simulink library "pwrsysVSrc"  (R2016a)
settings: Solver=VariableStepAuto  SolverMode=SingleTasking  StartTime=0.0  StopTime=10.0  RelTol=1e-3
undefined symbols (not defined in the file or in its folder): D1, Delta, DiscIntNeverNeededParam, ESS, fn, grid, Kp, PCC, Refmax, Refmin, sim, Tsm
undefined symbols (not defined in the file): exc, gov, Ts_c, turb, WT
libraries: powerlib x74, pwrsysBasic x1, sps_avr x1
settings Model: Creator=daniemot  LastModifiedBy=ericfa
settings DebuggingCC: SFUnexpectedBacktrackingDiag=error  SFNoUnconditionalDefaultTransitionDiag=error
settings GRTTargetCC: TargetLangStandard=C99 (ISO)  GeneratePreprocessorConditionals=Use local settings
settings ConfigComp: CovMetricSettings=dwe  CovHtmlReporting=off  CovSaveCumulativeToWorkspaceVar=off  CovSaveSingleToWorkspaceVar=off  CovExternalEMLEnable=on

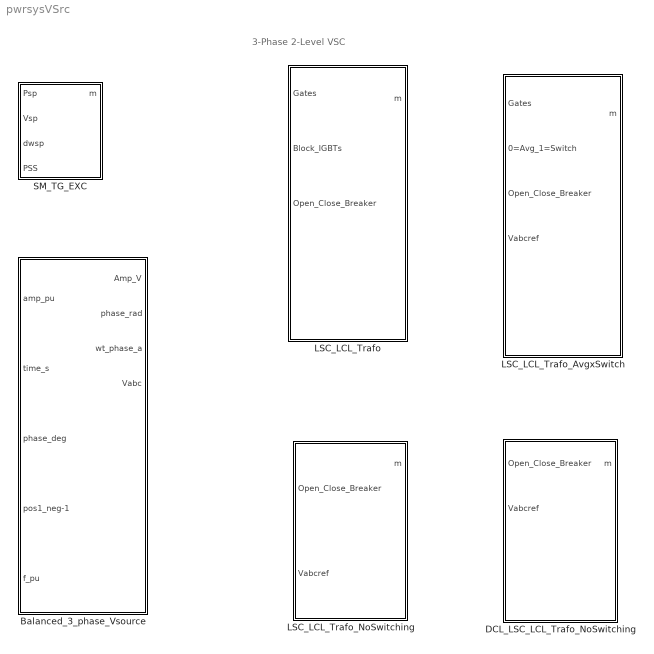
== system pwrsysVSrc ==
  note: 3-Phase 2-Level VSC
  Balanced_3_phase_Vsource : Subsystem  mask(Three-phase ideal voltage source){BaseAmp=1, fn=50}
      mask prompts: BaseAmp "Base phase-to-neutral amplitude [V]"; fn "Base frequency [Hz]"
      mask help:
      | Three-phase balanced ideal voltage source with neutral point not connected.
      | The voltage source can be connected in series with others.
      |
      | va [V] = amp_pu*BaseAmp*sin(2*pi*f_pu*fn*time + phase_deg*pi/180)
      | vb [V] = amp_pu*BaseAmp*sin(2*pi*f_pu*fn*time + phase_deg*pi/180 + Ph_b_sign*2*pi/3)
      | vc [V] = amp_pu*BaseAmp*sin(2*pi*f_pu*fn*time + phase_deg*pi/180 + Ph_c_sign*2*pi/3)
      |
      | If Pos1_Neg-1 = 1
      | 	Ph_b_sign = -1
      | 	Ph_c_sign = +1
      |
      | If Pos1_Neg-1 = -1
      | 	Ph_b_sign = +1
      | 	Ph_c_sign = -1
  DCL_LSC_LCL_Trafo_NoSwitching : Subsystem  mask(DCL + LSC + LCL + Trafo){Sn=WT.Sb, fn=fn, Uhv_ab=WT.ColSys.Ub, Uab=WT.LSC.Ub, lf2=WT.LSC.lf2, rf2=WT.LSC.rf2, Lf1=WT.LSC.Lf1, Rf1=WT.LSC.Rf1, Cf=WT.LSC.Cf, Rc=WT.LSC.Rc, Cdc=WT.LSC.Cf, Udc0=WT.LSC.Cf, Tsm=Tsm, Tstart=WT.LSC.Rc}
      mask prompts: Sn "Rated apparent power [VA]"; fn "Rated frequency [Hz]"; Uhv_ab "Trafo HV rated line voltage [V]"; Uab "Trafo LV rated line voltage [V]"; lf2 "Trafo short-circuit inductance, lf2 [pu]"; rf2 "Trafo short-circuit resistance, rf2 [pu]"; Lf1 "Inverter side inductande, Lf1 [H]"; Rf1 "Inverter side parasitic resistance, Rf1 [Ohm]"; Cf "Shunt branch capacitance, Cf [F]"; Rc "Shunt branch damping resistance, Rc [Ohm]"; Cdc "DC-link shunt capacitance, Cdc [F]"; Udc0 "DC-link initial voltage [V]"; Tsm "Measurement sampling time [s]"; Tstart "Start time [s]"
      mask help:
      | DC Link + Line-side converter + LCL filter + Transformer
      |
      | DCL: current sources
      | 	Cdc: shunt capacitor of DC-link
      |
      | LSC: voltage source
      | 	fpwm: PWM frequency
      | LCL:
      | 	Lf1 + Rf1: inverter side reactor
      | 	Cf + Rc: shunt capacitor and damping resistor
      | 	Lf2 + Rf2: transformer short circuit inductance and resistance
      |
      | Transformer:	Y d1
      | 	HV: Y ungrounded
      | 	LV: delta
      |
      | High resistive grounding on LV side of tranformer (0.001W)
  LSC_LCL_Trafo : Subsystem  mask(LSC + LCL + Trafo){Sn=WT.Sb, fn=fn, Uhv_ab=WT.ColSys.Ub, Uab=WT.LSC.Ub, lf2=WT.LSC.lf2, rf2=WT.LSC.rf2, Lf1=WT.LSC.Lf1, Rf1=WT.LSC.Rf1, Cf=WT.LSC.Cf, Rc=WT.LSC.Rc}
      mask prompts: Sn "Rated apparent power [VA]"; fn "Rated frequency [Hz]"; Uhv_ab "Trafo HV rated line voltage [V]"; Uab "Trafo LV rated line voltage [V]"; lf2 "Trafo short-circuit inductance, lf2 [pu]"; rf2 "Trafo short-circuit resistance, rf2 [pu]"; Lf1 "Inverter side inductande, Lf1 [H]"; Rf1 "Inverter side parasitic resistance, Rf1 [Ohm]"; Cf "Shunt branch capacitance, Cf [F]"; Rc "Shunt branch damping resistance, Rc [Ohm]"
      mask help:
      | Line side converter + LCL filter + Transformer
      |
      | LSC: switching devices
      | LCL:
      | 	Lf1 + Rf1: inverter side reactor
      | 	Cf + Rc: shunt capacitor and damping resistor
      | 	Lf2 + Rf2: transformer short circuit inductance and resistance
      |
      | Transformer:	Y d1
      | 	HV: Y ungrounded
      | 	LV: delta
      |
      | High resistive grounding on LV side of tranformer (0.001W)
  LSC_LCL_Trafo_AvgxSwitch : Subsystem  mask(LSC + LCL + Trafo){Sn=WT.Sb, fn=fn, Uhv_ab=WT.ColSys.Ub, Uab=WT.LSC.Ub, lf2=WT.LSC.lf2, rf2=WT.LSC.rf2, Lf1=WT.LSC.Lf1, Rf1=WT.LSC.Rf1, Cf=WT.LSC.Cf, Rc=WT.LSC.Rc}
      mask prompts: Sn "Rated apparent power [VA]"; fn "Rated frequency [Hz]"; Uhv_ab "Trafo HV rated line voltage [V]"; Uab "Trafo LV rated line voltage [V]"; lf2 "Trafo short-circuit inductance, lf2 [pu]"; rf2 "Trafo short-circuit resistance, rf2 [pu]"; Lf1 "Inverter side inductande, Lf1 [H]"; Rf1 "Inverter side parasitic resistance, Rf1 [Ohm]"; Cf "Shunt branch capacitance, Cf [F]"; Rc "Shunt branch damping resistance, Rc [Ohm]"
      mask help:
      | Line side converter + LCL filter + Transformer
      |
      | LSC: switching devices
      | LCL:
      | 	Lf1 + Rf1: inverter side reactor
      | 	Cf + Rc: shunt capacitor and damping resistor
      | 	Lf2 + Rf2: transformer short circuit inductance and resistance
      |
      | Transformer:	Y d1
      | 	HV: Y ungrounded
      | 	LV: delta
      |
      | High resistive grounding on LV side of tranformer (0.001W)
  LSC_LCL_Trafo_NoSwitching : Subsystem  mask(LSC + LCL + Trafo){Sn=WT.Sb, fn=fn, Uhv_ab=WT.ColSys.Ub, Uab=WT.LSC.Ub, lf2=WT.LSC.lf2, rf2=WT.LSC.rf2, Lf1=WT.LSC.Lf1, Rf1=WT.LSC.Rf1, Cf=WT.LSC.Cf, Rc=WT.LSC.Rc}
      mask prompts: Sn "Rated apparent power [VA]"; fn "Rated frequency [Hz]"; Uhv_ab "Trafo HV rated line voltage [V]"; Uab "Trafo LV rated line voltage [V]"; lf2 "Trafo short-circuit inductance, lf2 [pu]"; rf2 "Trafo short-circuit resistance, rf2 [pu]"; Lf1 "Inverter side inductande, Lf1 [H]"; Rf1 "Inverter side parasitic resistance, Rf1 [Ohm]"; Cf "Shunt branch capacitance, Cf [F]"; Rc "Shunt branch damping resistance, Rc [Ohm]"
      mask help:
      | Line side converter + LCL filter + Transformer
      |
      | LSC: switching devices
      | LCL:
      | 	Lf1 + Rf1: inverter side reactor
      | 	Cf + Rc: shunt capacitor and damping resistor
      | 	Lf2 + Rf2: transformer short circuit inductance and resistance
      |
      | Transformer:	Y d1
      | 	HV: Y ungrounded
      | 	LV: delta
      |
      | High resistive grounding on LV side of tranformer (0.001W)
  SM_TG_EXC : Subsystem  SystemSampleTime=10*sim.tStep  mask(Synchronous machine with governor and exciter){SMVn=sm.Vn, SMPn=sm.Sn, SMcosphi=sm.cosphi, SMfn=sm.fn, SMp=sm.p, SMM=sm.M, SMsat=sm.sat, SMXd=sm.Xd, SMXdp=sm.Xdp, SMXdpp=sm.Xdpp, SMXq=sm.Xq, SMXqpp=sm.Xqpp, SMXl=sm.Xl, SMRs=sm.Rs, SMTdpSC=sm.TdpSC, SMTdppSC=sm.TdppSC, SMTqppSC=sm.TqppSC, TurbT=turb.T, Ts=Ts_c, GovKp=gov.Kp, GovKd=gov.Kd, GovTr=gov.Tr, GovFlp=gov.flp, GovDB=gov.DB, ExcTr=exc.Tr, ExcKa=exc.Ka, ExcVRMax=exc.VRmax, ExcVRMin=exc.VRmin, ExcKf=exc.Kf, ExcTf=exc.Tf, ExcTb=exc.Tb, ExcTc=exc.Tc, ExcTb1=exc.Tb1, ExcTc1=exc.Tc1, TurbP0=turb.P0, SMVt0=sm.Vt0, SMEfd0=sm.Efd0, SMdw0=sm.dw0, SMth0=sm.th0, SMphi0=sm.phi0}
      mask prompts: SMVn "Voltage [V]"; SMPn "Apparent power [VA]"; SMcosphi "Power factor"; SMfn "Frequency [Hz]"; SMp "Pairs of poles"; SMM "Inertia constant [s]"; SMsat "Saturation curve in pu - [ifd; vt]"; SMXd "d-axis steady-state"; SMXdp "d-axis transient"; SMXdpp "d-axis subtransient"; SMXq "q-axis steady-state"; SMXqpp "q-axis subtransient"; SMXl "Leakage"; SMRs "Stator (armature) resistance"; SMTdpSC "d-axis transient time"; SMTdppSC "d-axis subtransient time"; SMTqppSC "q-axis subtransient time"; TurbT "Equivalent first-order delay [s]"; Ts "Sample time [s]"; GovKp "Permanent droop (primary control)"; GovKd "Transient droop (primary control)"; GovTr "Reset time transient droop (primary control)"; GovFlp "Low-pass frequency [Hz]"; GovDB "Deadband [pu]"; ExcTr "Input filter time constant [s]"; ExcKa "Proportional gain"; ExcVRMax "Maximum output [pu]"; ExcVRMin "Minimum output [pu]"; ExcKf "Rate feedback (derivative) gain"; ExcTf "Rate feedback (reset) time [s]"; ExcTb "1st lag time constant [s]"; ExcTc "1st lead time constant [s]"; ExcTb1 "2nd lag time constant [s]"; ExcTc1 "2nd lead time constant [s]"; TurbP0 "Turbine output [pu]"; SMVt0 "Stator voltage [pu]"; SMEfd0 "Field voltage [pu]"; SMdw0 "dw [%]"; SMth0 "theta [deg]"; SMphi0 "phi [deg]"
      mask help:
      | Synchronous machine + Generic Turbine Governor + IEEE ST1A Exciter
      |
      | This block is built using elements of the Simscape Specialized Power Systems library.
      |
      | Inputs:
      | Psp - Active power (P) setpoint in pu.
      |     Feed-forwarded to the turbine governor's Pxf droop controller. For precise P control, implement an external P controller.
      |
      | Vsp - RMS average voltage in pu.
      |     Connected to the Vref input of the IEEE ST1A Exciter.
      |
      | PSS - PSS contribution in pu.
      |     Connected to the Vstab input of the IEEE ST1A Exciter. Implement the PSS control loop externally.

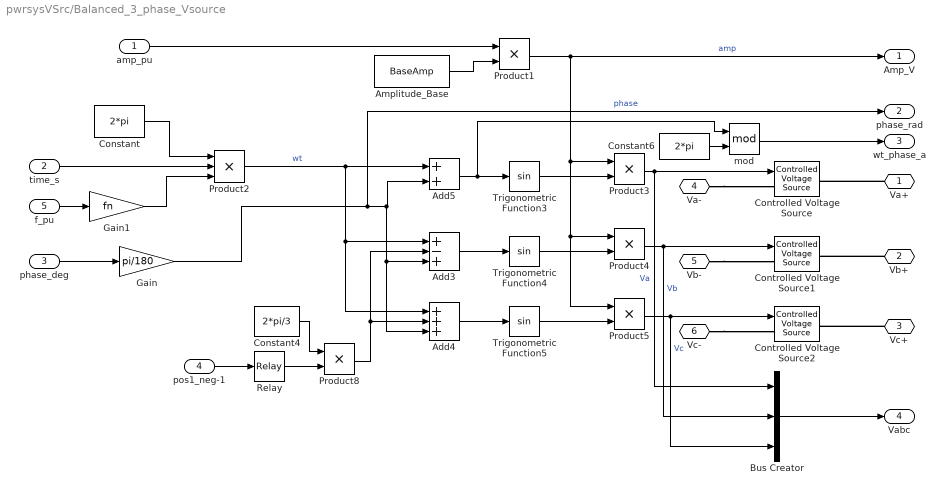
== system pwrsysVSrc/Balanced_3_phase_Vsource ==
  amp_pu : Inport
  time_s : Inport  Port=2
  phase_deg : Inport  Port=3
  pos1_neg-1 : Inport  Port=4
  f_pu : Inport  Port=5
  Add3 : Sum  Inputs=+-+
  Add4 : Sum  Inputs=+++
  Add5 : Sum
  Amplitude_Base : Constant  Value=BaseAmp
  Bus Creator : BusCreator  Inputs=3
  Constant : Constant  Value=2*pi
  Constant4 : Constant  Value=2*pi/3
  Constant6 : Constant  Value=2*pi
  Controlled Voltage Source : powerlib/Electrical Sources/Controlled Voltage Source  Initialize=off  Source_Type=AC  Amplitude=ESS.LSC.Ub*(2/3)^0.5  Phase=0  Frequency=PCC.fn  Measurements=None
  Controlled Voltage Source1 : powerlib/Electrical Sources/Controlled Voltage Source  Initialize=off  Source_Type=AC  Amplitude=ESS.LSC.Ub*(2/3)^0.5  Phase=-120  Frequency=PCC.fn  Measurements=None
  Controlled Voltage Source2 : powerlib/Electrical Sources/Controlled Voltage Source  Initialize=off  Source_Type=AC  Amplitude=ESS.LSC.Ub*(2/3)^0.5  Phase=120  Frequency=PCC.fn  Measurements=None
  Gain : Gain  Gain=pi/180
  Gain1 : Gain  Gain=fn
  Product{1,3..5,8} (5 alike) : Product
  Product2 : Product  Inputs=3
  Relay : Relay  OnSwitchValue=0  OffSwitchValue=-0.1  OffOutputValue=-1
  Trigonometric Function3 : Trigonometry
  Trigonometric Function4 : Trigonometry
  Trigonometric Function5 : Trigonometry
  mod : Math  Operator=mod  SaturateOnIntegerOverflow=on
  Va+ : PMIOPort  Port=1  Side=Right
  Vb+ : PMIOPort  Port=2  Side=Right
  Vc+ : PMIOPort  Port=3  Side=Right
  Va- : PMIOPort  Port=4  Side=Right
  Vb- : PMIOPort  Port=5  Side=Right
  Vc- : PMIOPort  Port=6  Side=Right
  Amp_V : Outport
  phase_rad : Outport  Port=2
  wt_phase_a : Outport  Port=3
  Vabc : Outport  Port=4
  wires:
  Add4/1 -> Trigonometric Function5/1
  Gain/1 -> phase_rad/1, Add4/3, Add3/3, Add5/2  "phase"
  Add3/1 -> Trigonometric Function4/1
  pos1_neg-1/1 -> Relay/1
  Product3/1 -> Bus Creator/1, Controlled Voltage Source/1  "Va"
  amp_pu/1 -> Product1/1
  Product8/1 -> Add3/2, Add4/2
  Product5/1 -> Bus Creator/3, Controlled Voltage Source2/1  "Vc"
  Product4/1 -> Bus Creator/2, Controlled Voltage Source1/1  "Vb"
  Amplitude_Base/1 -> Product1/2
  Constant4/1 -> Product8/1
  Product1/1 -> Product5/1, Product4/1, Product3/1, Amp_V/1  "amp"
  Relay/1 -> Product8/2
  Trigonometric Function3/1 -> Product3/2
  Product2/1 -> Add5/1, Add4/1, Add3/1  "wt"
  Trigonometric Function5/1 -> Product5/2
  Add5/1 -> mod/1, Trigonometric Function3/1
  Trigonometric Function4/1 -> Product4/2
  phase_deg/1 -> Gain/1
  time_s/1 -> Product2/2
  Constant/1 -> Product2/1
  f_pu/1 -> Gain1/1
  Gain1/1 -> Product2/3
  Bus Creator/1 -> Vabc/1
  Constant6/1 -> mod/2
  mod/1 -> wt_phase_a/1
  connections:
  Vb+/RConn1 -- Controlled Voltage Source1/RConn1
  Vc+/RConn1 -- Controlled Voltage Source2/RConn1
  Va+/RConn1 -- Controlled Voltage Source/RConn1
  Va-/RConn1 -- Controlled Voltage Source/LConn1
  Vb-/RConn1 -- Controlled Voltage Source1/LConn1
  Vc-/RConn1 -- Controlled Voltage Source2/LConn1

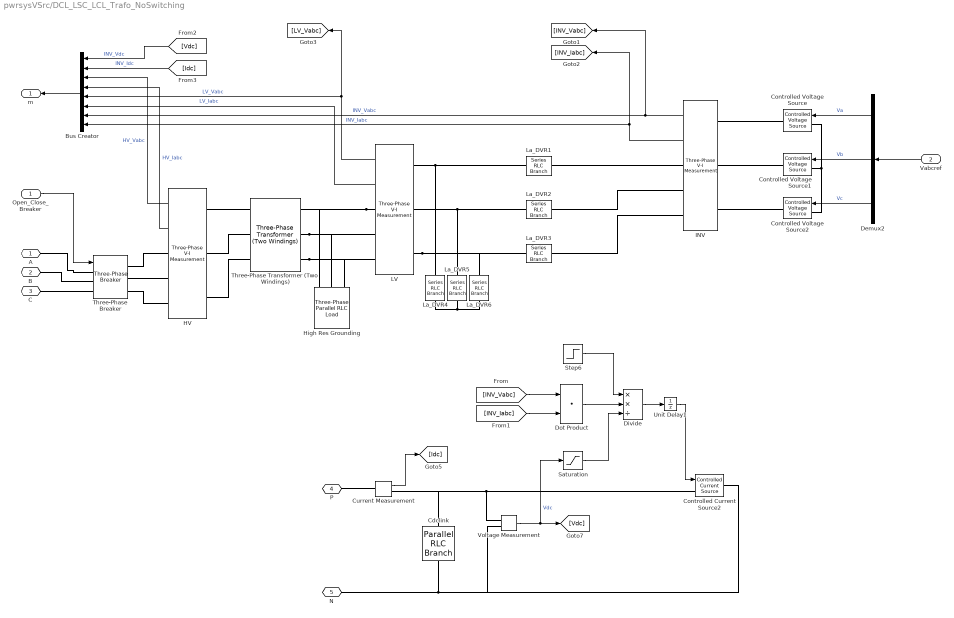
== system pwrsysVSrc/DCL_LSC_LCL_Trafo_NoSwitching ==
  Open_Close_Breaker : Inport
  Vabcref : Inport  Port=2
  Bus Creator : BusCreator  Inputs=8
  Cdclink : powerlib/Elements/Parallel RLC Branch  LConnTagsString=a  RConnTagsString=__new0  BranchType=RC  Resistance=1e6  Inductance=0  SetiL0=off  InitialCurrent=0  Capacitance=Cdc  Setx0=on  InitialVoltage=Udc0  Measurements=None
  Controlled Current Source2 : powerlib/Electrical Sources/Controlled Current Source  Initialize=on  Source_Type=DC  Amplitude=0  Phase=0  Frequency=50  Measurements=None
  Controlled Voltage Source : powerlib/Electrical Sources/Controlled Voltage Source  Initialize=on  Source_Type=AC  Amplitude=Uab*(2/3)^0.5  Phase=30  Frequency=fn  Measurements=None
  Controlled Voltage Source1 : powerlib/Electrical Sources/Controlled Voltage Source  Initialize=on  Source_Type=AC  Amplitude=Uab*(2/3)^0.5  Phase=30-120  Frequency=fn  Measurements=None
  Controlled Voltage Source2 : powerlib/Electrical Sources/Controlled Voltage Source  Initialize=on  Source_Type=AC  Amplitude=Uab*(2/3)^0.5  Phase=30+120  Frequency=fn  Measurements=None
  Current Measurement : powerlib/Measurements/Current Measurement  PhasorSimulation=off  OutputType=Complex  PSBequivalent=0
  Demux2 : Demux  Outputs=3
  Divide : Product  Inputs=**/
  Dot Product : DotProduct  InputSameDT=on  OutDataTypeStr=Inherit: Inherit via internal rule
  HV : powerlib/Measurements/Three-Phase V-I Measurement  VoltageMeasurement=phase-to-ground  SetLabelV=off  LabelV=vgrid  Vpu=off  VpuLL=off  CurrentMeasurement=yes  SetLabelI=off  LabelI=igrid  Ipu=off  Pbase=sn  Vbase=uab  OutputType=Complex  PhasorSimulation=off  PSBequivalent=0
  High Res Grounding : powerlib/Elements/Three-Phase Parallel RLC Load  LConnTagsString=A|B|C  Configuration=Y (grounded)  NominalVoltage=Uab  Vabc=[1e3 1e3 1e3]  Vabcp=[1e3 1e3 1e3]  NominalFrequency=fn  UnbalancedPower=off  ActivePower=0.001  InductivePower=0  CapacitivePower=0  Pabc=[10e3 9e3 11e3]  QLabc=[100 90 110]  QCabc=[100 90 110]  Pabcp=[10e3 9e3 11e3]  QLabcp=[100 90 110]  QCabcp=[100 90 110]  Measurements=None  LoadType=constant Z
  INV : powerlib/Measurements/Three-Phase V-I Measurement  VoltageMeasurement=phase-to-ground  SetLabelV=off  LabelV=vconv  Vpu=off  VpuLL=off  CurrentMeasurement=yes  SetLabelI=off  LabelI=iconv  Ipu=off  Pbase=sn  Vbase=uab  OutputType=Complex  PhasorSimulation=off  PSBequivalent=0
  LV : powerlib/Measurements/Three-Phase V-I Measurement  VoltageMeasurement=phase-to-ground  SetLabelV=off  LabelV=vgrid  Vpu=off  VpuLL=off  CurrentMeasurement=yes  SetLabelI=off  LabelI=igrid  Ipu=off  Pbase=sn  Vbase=uab  OutputType=Complex  PhasorSimulation=off  PSBequivalent=0
  La_DVR1 : powerlib/Elements/Series RLC Branch  LConnTagsString=__new0  RConnTagsString=__new0  BranchType=RL  Resistance=Rf1  Inductance=Lf1  SetiL0=off  InitialCurrent=0  Capacitance=1.0  Setx0=off  InitialVoltage=0  Measurements=None
  La_DVR2 : powerlib/Elements/Series RLC Branch  LConnTagsString=__new0  RConnTagsString=__new0  BranchType=RL  Resistance=Rf1  Inductance=Lf1  SetiL0=off  InitialCurrent=0  Capacitance=1.0  Setx0=off  InitialVoltage=0  Measurements=None
  La_DVR3 : powerlib/Elements/Series RLC Branch  LConnTagsString=__new0  RConnTagsString=__new0  BranchType=RL  Resistance=Rf1  Inductance=Lf1  SetiL0=off  InitialCurrent=0  Capacitance=1.0  Setx0=off  InitialVoltage=0  Measurements=None
  La_DVR4 : powerlib/Elements/Series RLC Branch  LConnTagsString=__new0  RConnTagsString=__new0  BranchType=RC  Resistance=Rc  Inductance=Lf1  SetiL0=off  InitialCurrent=0  Capacitance=Cf  Setx0=off  InitialVoltage=0  Measurements=None
  La_DVR5 : powerlib/Elements/Series RLC Branch  LConnTagsString=__new0  RConnTagsString=__new0  BranchType=RC  Resistance=Rc  Inductance=Lf1  SetiL0=off  InitialCurrent=0  Capacitance=Cf  Setx0=off  InitialVoltage=0  Measurements=None
  La_DVR6 : powerlib/Elements/Series RLC Branch  LConnTagsString=__new0  RConnTagsString=__new0  BranchType=RC  Resistance=Rc  Inductance=Lf1  SetiL0=off  InitialCurrent=0  Capacitance=Cf  Setx0=off  InitialVoltage=0  Measurements=None
  Saturation : Saturate  UpperLimit=10*Uab*sqrt(2/3)  LowerLimit=0.01*Uab*sqrt(2/3)
  Step6 : Step  Time=Tstart  SampleTime=Tsm
  Three-Phase Transformer (Two Windings) : powerlib/Elements/Three-Phase Transformer (Two Windings)  Winding1Connection=Y  Winding2Connection=Delta (D1)  CoreType=Three-limb core (core-type)  SetSaturation=off  Hysteresis=off  DataFile='hysteresis'  SetInitialFlux=off  Measurements=None  UNITS=pu  NominalPower=[ Sn , fn ]  Winding1=[ Uhv_ab , rf2/2 , lf2/2 ]  Winding2=[ Uab , rf2/2 , lf2/2 ]  Rm=500  Lm=500  L0=0.5  Saturation=[ 0,0 ; 0.0024,1.2 ; 1.0,1.52 ]  InitialFluxes=[0 0 0]  MoreParameters=off  BreakLoop=off  DataType=off  TransfoNumber=1
  Three-Phase Breaker : powerlib/Elements/Three-Phase Breaker  InitialState=open  SwitchA=on  SwitchB=on  SwitchC=on  SwitchTimes="[1/60  5/60]"  External=on  BreakerResistance=0.01  SnubberResistance=1e6  SnubberCapacitance=1e9  Measurements=None
  Unit Delay1 : UnitDelay  SampleTime=Tsm
  Voltage Measurement : powerlib/Measurements/Voltage Measurement  PhasorSimulation=off  OutputType=Magnitude  PSBequivalent=0
  A : PMIOPort  Port=1  Side=Right
  B : PMIOPort  Port=2  Side=Right
  C : PMIOPort  Port=3  Side=Right
  P : PMIOPort  Port=4  Side=Left
  N : PMIOPort  Port=5  Side=Left
  m : Outport
  wires:
  HV/2 -> Bus Creator/4  "HV_Iabc"
  LV/1 -> [LV_Vabc], Bus Creator/5  "LV_Vabc"
  INV/1 -> [INV_Vabc], Bus Creator/7  "INV_Vabc"
  INV/2 -> [INV_Iabc], Bus Creator/8  "INV_Iabc"
  HV/1 -> Bus Creator/3  "HV_Vabc"
  LV/2 -> Bus Creator/6  "LV_Iabc"
  Bus Creator/1 -> m/1
  Open_Close_Breaker/1 -> Three-Phase Breaker/1
  Vabcref/1 -> Demux2/1
  Demux2/1 -> Controlled Voltage Source/1  "Va"
  Demux2/2 -> Controlled Voltage Source1/1  "Vb"
  Demux2/3 -> Controlled Voltage Source2/1  "Vc"
  Voltage Measurement/1 -> [Vdc], Saturation/1  "Vdc"
  Saturation/1 -> Divide/3
  Dot Product/1 -> Divide/2
  Divide/1 -> Unit Delay1/1
  [INV_Vabc] -> Dot Product/1
  [INV_Iabc] -> Dot Product/2
  [Vdc] -> Bus Creator/1  "INV_Vdc"
  [Idc] -> Bus Creator/2  "INV_Idc"
  Unit Delay1/1 -> Controlled Current Source2/1
  Step6/1 -> Divide/1
  Current Measurement/1 -> [Idc]
  connections:
  La_DVR1/LConn1 -- INV/RConn1
  LV/RConn1 -- Three-Phase Transformer (Two Windings)/RConn1 -- High Res Grounding/LConn1
  La_DVR1/RConn1 -- La_DVR4/RConn1 -- LV/LConn1
  Three-Phase Transformer (Two Windings)/LConn3 -- HV/LConn3
  Three-Phase Transformer (Two Windings)/RConn3 -- LV/RConn3 -- High Res Grounding/LConn3
  La_DVR2/RConn1 -- La_DVR5/RConn1 -- LV/LConn2
  Three-Phase Transformer (Two Windings)/LConn2 -- HV/LConn2
  Three-Phase Transformer (Two Windings)/RConn2 -- LV/RConn2 -- High Res Grounding/LConn2
  Three-Phase Transformer (Two Windings)/LConn1 -- HV/LConn1
  LV/LConn3 -- La_DVR3/RConn1 -- La_DVR6/RConn1
  La_DVR3/LConn1 -- INV/RConn3
  La_DVR5/LConn1 -- La_DVR6/LConn1 -- La_DVR4/LConn1
  La_DVR2/LConn1 -- INV/RConn2
  Three-Phase Breaker/LConn2 -- B/RConn1
  Three-Phase Breaker/RConn2 -- HV/RConn2
  HV/RConn3 -- Three-Phase Breaker/RConn3
  Three-Phase Breaker/LConn3 -- C/RConn1
  HV/RConn1 -- Three-Phase Breaker/RConn1
  Three-Phase Breaker/LConn1 -- A/RConn1
  Controlled Voltage Source2/LConn1 -- Controlled Voltage Source/LConn1 -- Controlled Voltage Source1/LConn1
  INV/LConn1 -- Controlled Voltage Source/RConn1
  Controlled Voltage Source1/RConn1 -- INV/LConn2
  Controlled Voltage Source2/RConn1 -- INV/LConn3
  Voltage Measurement/LConn2 -- Controlled Current Source2/RConn1 -- Cdclink/RConn1 -- N/RConn1
  Controlled Current Source2/LConn1 -- Current Measurement/RConn1 -- Cdclink/LConn1 -- Voltage Measurement/LConn1
  P/RConn1 -- Current Measurement/LConn1

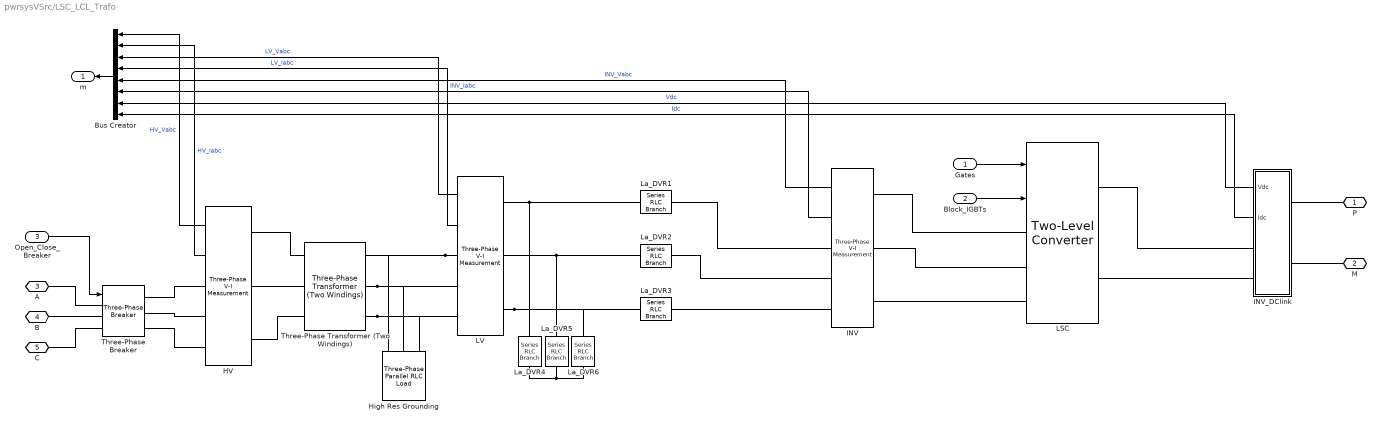
== system pwrsysVSrc/LSC_LCL_Trafo ==
  Gates : Inport
  Block_IGBTs : Inport  Port=2
  Open_Close_Breaker : Inport  Port=3
  Bus Creator : BusCreator  Inputs=8
  HV : powerlib/Measurements/Three-Phase V-I Measurement  VoltageMeasurement=phase-to-ground  SetLabelV=off  LabelV=vgrid  Vpu=off  VpuLL=off  CurrentMeasurement=yes  SetLabelI=off  LabelI=igrid  Ipu=off  Pbase=sn  Vbase=uab  OutputType=Complex  PhasorSimulation=off  PSBequivalent=0
  High Res Grounding : powerlib/Elements/Three-Phase Parallel RLC Load  LConnTagsString=A|B|C  Configuration=Y (grounded)  NominalVoltage=Uab  Vabc=[1e3 1e3 1e3]  Vabcp=[1e3 1e3 1e3]  NominalFrequency=fn  UnbalancedPower=off  ActivePower=0.001  InductivePower=0  CapacitivePower=0  Pabc=[10e3 9e3 11e3]  QLabc=[100 90 110]  QCabc=[100 90 110]  Pabcp=[10e3 9e3 11e3]  QLabcp=[100 90 110]  QCabcp=[100 90 110]  Measurements=None  LoadType=constant Z
  INV : powerlib/Measurements/Three-Phase V-I Measurement  VoltageMeasurement=phase-to-ground  SetLabelV=off  LabelV=vconv  Vpu=off  VpuLL=off  CurrentMeasurement=yes  SetLabelI=off  LabelI=iconv  Ipu=off  Pbase=sn  Vbase=uab  OutputType=Complex  PhasorSimulation=off  PSBequivalent=0
  INV_DClink : Subsystem
  LSC : powerlib/Power Electronics/Two-Level Converter  ModelType=Switching devices  Ron=1e-3  Rs=1e6  Cs=inf  Vforward=[ 0, 0 ]  Ron_Diode=1e-3  Rs_Diode=1e6  Cs_Diode=inf  Vf_Diode=1e-3  Rs_CurrentSource=inf
      settings: AttributesFormatString=%<ModelType>
  LV : powerlib/Measurements/Three-Phase V-I Measurement  VoltageMeasurement=phase-to-ground  SetLabelV=off  LabelV=vgrid  Vpu=off  VpuLL=off  CurrentMeasurement=yes  SetLabelI=off  LabelI=igrid  Ipu=off  Pbase=sn  Vbase=uab  OutputType=Complex  PhasorSimulation=off  PSBequivalent=0
  La_DVR1 : powerlib/Elements/Series RLC Branch  LConnTagsString=__new0  RConnTagsString=__new0  BranchType=RL  Resistance=Rf1  Inductance=Lf1  SetiL0=off  InitialCurrent=0  Capacitance=1.0  Setx0=off  InitialVoltage=0  Measurements=None
  La_DVR2 : powerlib/Elements/Series RLC Branch  LConnTagsString=__new0  RConnTagsString=__new0  BranchType=RL  Resistance=Rf1  Inductance=Lf1  SetiL0=off  InitialCurrent=0  Capacitance=1.0  Setx0=off  InitialVoltage=0  Measurements=None
  La_DVR3 : powerlib/Elements/Series RLC Branch  LConnTagsString=__new0  RConnTagsString=__new0  BranchType=RL  Resistance=Rf1  Inductance=Lf1  SetiL0=off  InitialCurrent=0  Capacitance=1.0  Setx0=off  InitialVoltage=0  Measurements=None
  La_DVR4 : powerlib/Elements/Series RLC Branch  LConnTagsString=__new0  RConnTagsString=__new0  BranchType=RC  Resistance=Rc  Inductance=Lf1  SetiL0=off  InitialCurrent=0  Capacitance=Cf  Setx0=off  InitialVoltage=0  Measurements=None
  La_DVR5 : powerlib/Elements/Series RLC Branch  LConnTagsString=__new0  RConnTagsString=__new0  BranchType=RC  Resistance=Rc  Inductance=Lf1  SetiL0=off  InitialCurrent=0  Capacitance=Cf  Setx0=off  InitialVoltage=0  Measurements=None
  La_DVR6 : powerlib/Elements/Series RLC Branch  LConnTagsString=__new0  RConnTagsString=__new0  BranchType=RC  Resistance=Rc  Inductance=Lf1  SetiL0=off  InitialCurrent=0  Capacitance=Cf  Setx0=off  InitialVoltage=0  Measurements=None
  Three-Phase Transformer (Two Windings) : powerlib/Elements/Three-Phase Transformer (Two Windings)  Winding1Connection=Y  Winding2Connection=Delta (D1)  CoreType=Three-limb core (core-type)  SetSaturation=off  Hysteresis=off  DataFile='hysteresis'  SetInitialFlux=off  Measurements=None  UNITS=pu  NominalPower=[ Sn , fn ]  Winding1=[ Uhv_ab , rf2/2 , lf2/2 ]  Winding2=[ Uab , rf2/2 , lf2/2 ]  Rm=500  Lm=500  L0=0.5  Saturation=[ 0,0 ; 0.0024,1.2 ; 1.0,1.52 ]  InitialFluxes=[0 0 0]  MoreParameters=off  BreakLoop=off  DataType=off  TransfoNumber=1
  Three-Phase Breaker : powerlib/Elements/Three-Phase Breaker  InitialState=open  SwitchA=on  SwitchB=on  SwitchC=on  SwitchTimes="[1/60  5/60]"  External=on  BreakerResistance=0.01  SnubberResistance=1e6  SnubberCapacitance=1e9  Measurements=None
  "\tP" : PMIOPort  Port=1  Side=Left
  M : PMIOPort  Port=2  Side=Left
  A : PMIOPort  Port=3  Side=Right
  B : PMIOPort  Port=4  Side=Right
  C : PMIOPort  Port=5  Side=Right
  m : Outport
  wires:
  HV/2 -> Bus Creator/2  "HV_Iabc"
  LV/1 -> Bus Creator/3  "LV_Vabc"
  INV/1 -> Bus Creator/5  "INV_Vabc"
  INV_DClink/2(Idc) -> Bus Creator/8  "Idc"
  INV/2 -> Bus Creator/6  "INV_Iabc"
  Block_IGBTs/1 -> LSC/2
  INV_DClink/1(Vdc) -> Bus Creator/7  "Vdc"
  HV/1 -> Bus Creator/1  "HV_Vabc"
  LV/2 -> Bus Creator/4  "LV_Iabc"
  Bus Creator/1 -> m/1
  Gates/1 -> LSC/1
  Open_Close_Breaker/1 -> Three-Phase Breaker/1
  connections:
  La_DVR1/LConn1 -- INV/RConn1
  LV/RConn1 -- Three-Phase Transformer (Two Windings)/RConn1 -- High Res Grounding/LConn1
  La_DVR1/RConn1 -- La_DVR4/RConn1 -- LV/LConn1
  LSC/LConn3 -- INV/LConn3
  Three-Phase Transformer (Two Windings)/LConn3 -- HV/LConn3
  LSC/LConn2 -- INV/LConn2
  Three-Phase Transformer (Two Windings)/RConn3 -- LV/RConn3 -- High Res Grounding/LConn3
  La_DVR2/RConn1 -- La_DVR5/RConn1 -- LV/LConn2
  Three-Phase Transformer (Two Windings)/LConn2 -- HV/LConn2
  LSC/RConn2 -- INV_DClink/RConn2
  LSC/LConn1 -- INV/LConn1
  LSC/RConn1 -- INV_DClink/RConn1
  Three-Phase Transformer (Two Windings)/RConn2 -- LV/RConn2 -- High Res Grounding/LConn2
  "\tP"/RConn1 -- INV_DClink/LConn1
  Three-Phase Transformer (Two Windings)/LConn1 -- HV/LConn1
  LV/LConn3 -- La_DVR3/RConn1 -- La_DVR6/RConn1
  La_DVR3/LConn1 -- INV/RConn3
  La_DVR5/LConn1 -- La_DVR6/LConn1 -- La_DVR4/LConn1
  La_DVR2/LConn1 -- INV/RConn2
  INV_DClink/LConn2 -- M/RConn1
  Three-Phase Breaker/LConn2 -- B/RConn1
  Three-Phase Breaker/RConn2 -- HV/RConn2
  HV/RConn3 -- Three-Phase Breaker/RConn3
  Three-Phase Breaker/LConn3 -- C/RConn1
  HV/RConn1 -- Three-Phase Breaker/RConn1
  Three-Phase Breaker/LConn1 -- A/RConn1

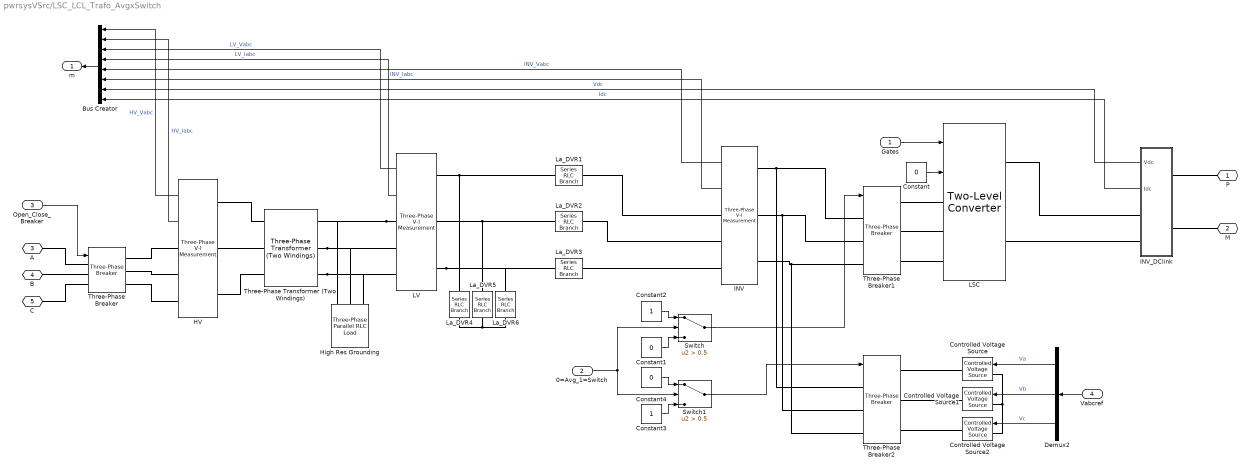
== system pwrsysVSrc/LSC_LCL_Trafo_AvgxSwitch ==
  Gates : Inport
  0=Avg_1=Switch : Inport  Port=2
  Open_Close_Breaker : Inport  Port=3
  Vabcref : Inport  Port=4
  Bus Creator : BusCreator  Inputs=8
  Constant : Constant  Value=0
  Constant1 : Constant  Value=0
  Constant2 : Constant
  Constant3 : Constant
  Constant4 : Constant  Value=0
  Controlled Voltage Source : powerlib/Electrical Sources/Controlled Voltage Source  Initialize=off  Source_Type=AC  Amplitude=ESS.LSC.Ub*(2/3)^0.5  Phase=0  Frequency=PCC.fn  Measurements=None
  Controlled Voltage Source1 : powerlib/Electrical Sources/Controlled Voltage Source  Initialize=off  Source_Type=AC  Amplitude=ESS.LSC.Ub*(2/3)^0.5  Phase=-120  Frequency=PCC.fn  Measurements=None
  Controlled Voltage Source2 : powerlib/Electrical Sources/Controlled Voltage Source  Initialize=off  Source_Type=AC  Amplitude=ESS.LSC.Ub*(2/3)^0.5  Phase=120  Frequency=PCC.fn  Measurements=None
  Demux2 : Demux  Outputs=3
  HV : powerlib/Measurements/Three-Phase V-I Measurement  VoltageMeasurement=phase-to-ground  SetLabelV=off  LabelV=vgrid  Vpu=off  VpuLL=off  CurrentMeasurement=yes  SetLabelI=off  LabelI=igrid  Ipu=off  Pbase=sn  Vbase=uab  OutputType=Complex  PhasorSimulation=off  PSBequivalent=0
  High Res Grounding : powerlib/Elements/Three-Phase Parallel RLC Load  LConnTagsString=A|B|C  Configuration=Y (grounded)  NominalVoltage=Uab  Vabc=[1e3 1e3 1e3]  Vabcp=[1e3 1e3 1e3]  NominalFrequency=fn  UnbalancedPower=off  ActivePower=0.001  InductivePower=0  CapacitivePower=0  Pabc=[10e3 9e3 11e3]  QLabc=[100 90 110]  QCabc=[100 90 110]  Pabcp=[10e3 9e3 11e3]  QLabcp=[100 90 110]  QCabcp=[100 90 110]  Measurements=None  LoadType=constant Z
  INV : powerlib/Measurements/Three-Phase V-I Measurement  VoltageMeasurement=phase-to-ground  SetLabelV=off  LabelV=vconv  Vpu=off  VpuLL=off  CurrentMeasurement=yes  SetLabelI=off  LabelI=iconv  Ipu=off  Pbase=sn  Vbase=uab  OutputType=Complex  PhasorSimulation=off  PSBequivalent=0
  INV_DClink : Subsystem
  LSC : powerlib/Power Electronics/Two-Level Converter  ModelType=Switching devices  Ron=1e-3  Rs=1e6  Cs=inf  Vforward=[ 0, 0 ]  Ron_Diode=1e-3  Rs_Diode=1e6  Cs_Diode=inf  Vf_Diode=1e-3  Rs_CurrentSource=inf
      settings: AttributesFormatString=%<ModelType>
  LV : powerlib/Measurements/Three-Phase V-I Measurement  VoltageMeasurement=phase-to-ground  SetLabelV=off  LabelV=vgrid  Vpu=off  VpuLL=off  CurrentMeasurement=yes  SetLabelI=off  LabelI=igrid  Ipu=off  Pbase=sn  Vbase=uab  OutputType=Complex  PhasorSimulation=off  PSBequivalent=0
  La_DVR1 : powerlib/Elements/Series RLC Branch  LConnTagsString=__new0  RConnTagsString=__new0  BranchType=RL  Resistance=Rf1  Inductance=Lf1  SetiL0=off  InitialCurrent=0  Capacitance=1.0  Setx0=off  InitialVoltage=0  Measurements=None
  La_DVR2 : powerlib/Elements/Series RLC Branch  LConnTagsString=__new0  RConnTagsString=__new0  BranchType=RL  Resistance=Rf1  Inductance=Lf1  SetiL0=off  InitialCurrent=0  Capacitance=1.0  Setx0=off  InitialVoltage=0  Measurements=None
  La_DVR3 : powerlib/Elements/Series RLC Branch  LConnTagsString=__new0  RConnTagsString=__new0  BranchType=RL  Resistance=Rf1  Inductance=Lf1  SetiL0=off  InitialCurrent=0  Capacitance=1.0  Setx0=off  InitialVoltage=0  Measurements=None
  La_DVR4 : powerlib/Elements/Series RLC Branch  LConnTagsString=__new0  RConnTagsString=__new0  BranchType=RC  Resistance=Rc  Inductance=Lf1  SetiL0=off  InitialCurrent=0  Capacitance=Cf  Setx0=off  InitialVoltage=0  Measurements=None
  La_DVR5 : powerlib/Elements/Series RLC Branch  LConnTagsString=__new0  RConnTagsString=__new0  BranchType=RC  Resistance=Rc  Inductance=Lf1  SetiL0=off  InitialCurrent=0  Capacitance=Cf  Setx0=off  InitialVoltage=0  Measurements=None
  La_DVR6 : powerlib/Elements/Series RLC Branch  LConnTagsString=__new0  RConnTagsString=__new0  BranchType=RC  Resistance=Rc  Inductance=Lf1  SetiL0=off  InitialCurrent=0  Capacitance=Cf  Setx0=off  InitialVoltage=0  Measurements=None
  Switch : Switch  Criteria=u2 > Threshold  Threshold=0.5
  Switch1 : Switch  Criteria=u2 > Threshold  Threshold=0.5
  Three-Phase Transformer (Two Windings) : powerlib/Elements/Three-Phase Transformer (Two Windings)  Winding1Connection=Y  Winding2Connection=Delta (D1)  CoreType=Three-limb core (core-type)  SetSaturation=off  Hysteresis=off  DataFile='hysteresis'  SetInitialFlux=off  Measurements=None  UNITS=pu  NominalPower=[ Sn , fn ]  Winding1=[ Uhv_ab , rf2/2 , lf2/2 ]  Winding2=[ Uab , rf2/2 , lf2/2 ]  Rm=500  Lm=500  L0=0.5  Saturation=[ 0,0 ; 0.0024,1.2 ; 1.0,1.52 ]  InitialFluxes=[0 0 0]  MoreParameters=off  BreakLoop=off  DataType=off  TransfoNumber=1
  Three-Phase Breaker : powerlib/Elements/Three-Phase Breaker  InitialState=open  SwitchA=on  SwitchB=on  SwitchC=on  SwitchTimes="[1/60  5/60]"  External=on  BreakerResistance=0.01  SnubberResistance=1e6  SnubberCapacitance=1e9  Measurements=None
  Three-Phase Breaker1 : powerlib/Elements/Three-Phase Breaker  InitialState=open  SwitchA=on  SwitchB=on  SwitchC=on  SwitchTimes="[1/60  5/60]"  External=on  BreakerResistance=0.000000000001  SnubberResistance=1e10  SnubberCapacitance=inf  Measurements=None
  Three-Phase Breaker2 : powerlib/Elements/Three-Phase Breaker  InitialState=open  SwitchA=on  SwitchB=on  SwitchC=on  SwitchTimes="[1/60  5/60]"  External=on  BreakerResistance=0.000000000001  SnubberResistance=1e10  SnubberCapacitance=inf  Measurements=None
  "\tP" : PMIOPort  Port=1  Side=Left
  M : PMIOPort  Port=2  Side=Left
  A : PMIOPort  Port=3  Side=Right
  B : PMIOPort  Port=4  Side=Right
  C : PMIOPort  Port=5  Side=Right
  m : Outport
  wires:
  HV/2 -> Bus Creator/2  "HV_Iabc"
  LV/1 -> Bus Creator/3  "LV_Vabc"
  INV/1 -> Bus Creator/5  "INV_Vabc"
  INV_DClink/2(Idc) -> Bus Creator/8  "Idc"
  INV/2 -> Bus Creator/6  "INV_Iabc"
  INV_DClink/1(Vdc) -> Bus Creator/7  "Vdc"
  HV/1 -> Bus Creator/1  "HV_Vabc"
  LV/2 -> Bus Creator/4  "LV_Iabc"
  Bus Creator/1 -> m/1
  Gates/1 -> LSC/1
  Open_Close_Breaker/1 -> Three-Phase Breaker/1
  Vabcref/1 -> Demux2/1
  Demux2/1 -> Controlled Voltage Source/1  "Va"
  Demux2/2 -> Controlled Voltage Source1/1  "Vb"
  Demux2/3 -> Controlled Voltage Source2/1  "Vc"
  Constant/1 -> LSC/2
  Constant1/1 -> Switch/3
  Constant2/1 -> Switch/1
  Switch/1 -> Three-Phase Breaker1/1
  Constant4/1 -> Switch1/1
  Constant3/1 -> Switch1/3
  Switch1/1 -> Three-Phase Breaker2/1
  0=Avg_1=Switch/1 -> Switch1/2, Switch/2
  connections:
  La_DVR1/LConn1 -- INV/RConn1
  LV/RConn1 -- Three-Phase Transformer (Two Windings)/RConn1 -- High Res Grounding/LConn1
  La_DVR1/RConn1 -- La_DVR4/RConn1 -- LV/LConn1
  LSC/LConn3 -- Three-Phase Breaker1/RConn3
  Three-Phase Transformer (Two Windings)/LConn3 -- HV/LConn3
  LSC/LConn2 -- Three-Phase Breaker1/RConn2
  Three-Phase Transformer (Two Windings)/RConn3 -- LV/RConn3 -- High Res Grounding/LConn3
  La_DVR2/RConn1 -- La_DVR5/RConn1 -- LV/LConn2
  Three-Phase Transformer (Two Windings)/LConn2 -- HV/LConn2
  LSC/RConn2 -- INV_DClink/RConn2
  LSC/LConn1 -- Three-Phase Breaker1/RConn1
  LSC/RConn1 -- INV_DClink/RConn1
  Three-Phase Transformer (Two Windings)/RConn2 -- LV/RConn2 -- High Res Grounding/LConn2
  "\tP"/RConn1 -- INV_DClink/LConn1
  Three-Phase Transformer (Two Windings)/LConn1 -- HV/LConn1
  LV/LConn3 -- La_DVR3/RConn1 -- La_DVR6/RConn1
  La_DVR3/LConn1 -- INV/RConn3
  La_DVR5/LConn1 -- La_DVR6/LConn1 -- La_DVR4/LConn1
  La_DVR2/LConn1 -- INV/RConn2
  INV_DClink/LConn2 -- M/RConn1
  Three-Phase Breaker/LConn2 -- B/RConn1
  Three-Phase Breaker/RConn2 -- HV/RConn2
  HV/RConn3 -- Three-Phase Breaker/RConn3
  Three-Phase Breaker/LConn3 -- C/RConn1
  HV/RConn1 -- Three-Phase Breaker/RConn1
  Three-Phase Breaker/LConn1 -- A/RConn1
  Controlled Voltage Source2/LConn1 -- Controlled Voltage Source/LConn1 -- Controlled Voltage Source1/LConn1
  Three-Phase Breaker1/LConn1 -- Three-Phase Breaker2/LConn1 -- INV/LConn1
  Three-Phase Breaker1/LConn2 -- Three-Phase Breaker2/LConn2 -- INV/LConn2
  Three-Phase Breaker1/LConn3 -- Three-Phase Breaker2/LConn3 -- INV/LConn3
  Three-Phase Breaker2/RConn1 -- Controlled Voltage Source/RConn1
  Controlled Voltage Source1/RConn1 -- Three-Phase Breaker2/RConn2
  Controlled Voltage Source2/RConn1 -- Three-Phase Breaker2/RConn3

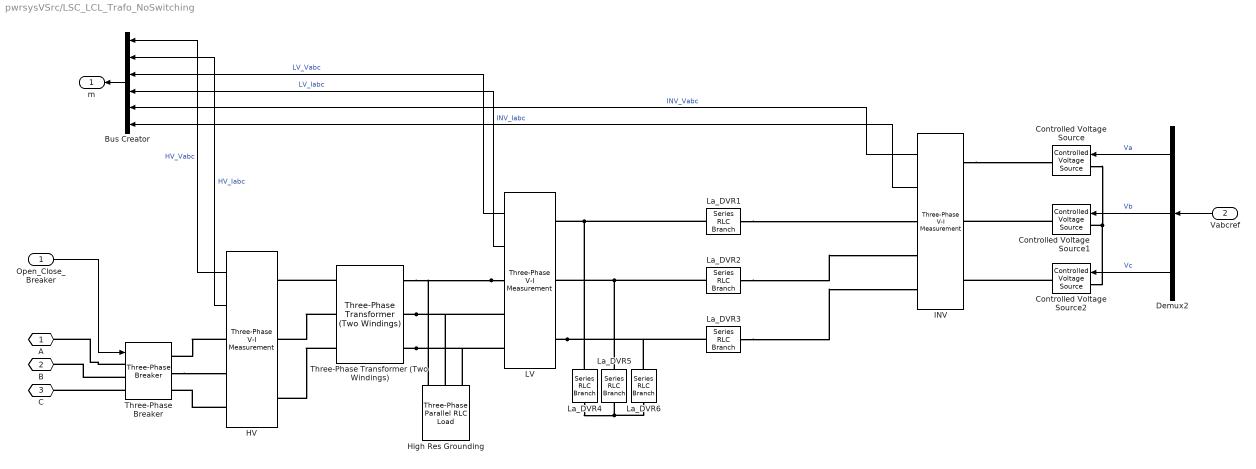
== system pwrsysVSrc/LSC_LCL_Trafo_NoSwitching ==
  Open_Close_Breaker : Inport
  Vabcref : Inport  Port=2
  Bus Creator : BusCreator  Inputs=6
  Controlled Voltage Source : powerlib/Electrical Sources/Controlled Voltage Source  Initialize=on  Source_Type=AC  Amplitude=Uab*(2/3)^0.5  Phase=30  Frequency=fn  Measurements=None
  Controlled Voltage Source1 : powerlib/Electrical Sources/Controlled Voltage Source  Initialize=on  Source_Type=AC  Amplitude=Uab*(2/3)^0.5  Phase=30-120  Frequency=fn  Measurements=None
  Controlled Voltage Source2 : powerlib/Electrical Sources/Controlled Voltage Source  Initialize=on  Source_Type=AC  Amplitude=Uab*(2/3)^0.5  Phase=30+120  Frequency=fn  Measurements=None
  Demux2 : Demux  Outputs=3
  HV : powerlib/Measurements/Three-Phase V-I Measurement  VoltageMeasurement=phase-to-ground  SetLabelV=off  LabelV=vgrid  Vpu=off  VpuLL=off  CurrentMeasurement=yes  SetLabelI=off  LabelI=igrid  Ipu=off  Pbase=sn  Vbase=uab  OutputType=Complex  PhasorSimulation=off  PSBequivalent=0
  High Res Grounding : powerlib/Elements/Three-Phase Parallel RLC Load  LConnTagsString=A|B|C  Configuration=Y (grounded)  NominalVoltage=Uab  Vabc=[1e3 1e3 1e3]  Vabcp=[1e3 1e3 1e3]  NominalFrequency=fn  UnbalancedPower=off  ActivePower=0.001  InductivePower=0  CapacitivePower=0  Pabc=[10e3 9e3 11e3]  QLabc=[100 90 110]  QCabc=[100 90 110]  Pabcp=[10e3 9e3 11e3]  QLabcp=[100 90 110]  QCabcp=[100 90 110]  Measurements=None  LoadType=constant Z
  INV : powerlib/Measurements/Three-Phase V-I Measurement  VoltageMeasurement=phase-to-ground  SetLabelV=off  LabelV=vconv  Vpu=off  VpuLL=off  CurrentMeasurement=yes  SetLabelI=off  LabelI=iconv  Ipu=off  Pbase=sn  Vbase=uab  OutputType=Complex  PhasorSimulation=off  PSBequivalent=0
  LV : powerlib/Measurements/Three-Phase V-I Measurement  VoltageMeasurement=phase-to-ground  SetLabelV=off  LabelV=vgrid  Vpu=off  VpuLL=off  CurrentMeasurement=yes  SetLabelI=off  LabelI=igrid  Ipu=off  Pbase=sn  Vbase=uab  OutputType=Complex  PhasorSimulation=off  PSBequivalent=0
  La_DVR1 : powerlib/Elements/Series RLC Branch  LConnTagsString=__new0  RConnTagsString=__new0  BranchType=RL  Resistance=Rf1  Inductance=Lf1  SetiL0=off  InitialCurrent=0  Capacitance=1.0  Setx0=off  InitialVoltage=0  Measurements=None
  La_DVR2 : powerlib/Elements/Series RLC Branch  LConnTagsString=__new0  RConnTagsString=__new0  BranchType=RL  Resistance=Rf1  Inductance=Lf1  SetiL0=off  InitialCurrent=0  Capacitance=1.0  Setx0=off  InitialVoltage=0  Measurements=None
  La_DVR3 : powerlib/Elements/Series RLC Branch  LConnTagsString=__new0  RConnTagsString=__new0  BranchType=RL  Resistance=Rf1  Inductance=Lf1  SetiL0=off  InitialCurrent=0  Capacitance=1.0  Setx0=off  InitialVoltage=0  Measurements=None
  La_DVR4 : powerlib/Elements/Series RLC Branch  LConnTagsString=__new0  RConnTagsString=__new0  BranchType=RC  Resistance=Rc  Inductance=Lf1  SetiL0=off  InitialCurrent=0  Capacitance=Cf  Setx0=off  InitialVoltage=0  Measurements=None
  La_DVR5 : powerlib/Elements/Series RLC Branch  LConnTagsString=__new0  RConnTagsString=__new0  BranchType=RC  Resistance=Rc  Inductance=Lf1  SetiL0=off  InitialCurrent=0  Capacitance=Cf  Setx0=off  InitialVoltage=0  Measurements=None
  La_DVR6 : powerlib/Elements/Series RLC Branch  LConnTagsString=__new0  RConnTagsString=__new0  BranchType=RC  Resistance=Rc  Inductance=Lf1  SetiL0=off  InitialCurrent=0  Capacitance=Cf  Setx0=off  InitialVoltage=0  Measurements=None
  Three-Phase Transformer (Two Windings) : powerlib/Elements/Three-Phase Transformer (Two Windings)  Winding1Connection=Y  Winding2Connection=Delta (D1)  CoreType=Three-limb core (core-type)  SetSaturation=off  Hysteresis=off  DataFile='hysteresis'  SetInitialFlux=off  Measurements=None  UNITS=pu  NominalPower=[ Sn , fn ]  Winding1=[ Uhv_ab , rf2/2 , lf2/2 ]  Winding2=[ Uab , rf2/2 , lf2/2 ]  Rm=500  Lm=500  L0=0.5  Saturation=[ 0,0 ; 0.0024,1.2 ; 1.0,1.52 ]  InitialFluxes=[0 0 0]  MoreParameters=off  BreakLoop=off  DataType=off  TransfoNumber=1
  Three-Phase Breaker : powerlib/Elements/Three-Phase Breaker  InitialState=open  SwitchA=on  SwitchB=on  SwitchC=on  SwitchTimes="[1/60  5/60]"  External=on  BreakerResistance=0.01  SnubberResistance=1e6  SnubberCapacitance=1e9  Measurements=None
  A : PMIOPort  Port=1  Side=Right
  B : PMIOPort  Port=2  Side=Right
  C : PMIOPort  Port=3  Side=Right
  m : Outport
  wires:
  HV/2 -> Bus Creator/2  "HV_Iabc"
  LV/1 -> Bus Creator/3  "LV_Vabc"
  INV/1 -> Bus Creator/5  "INV_Vabc"
  INV/2 -> Bus Creator/6  "INV_Iabc"
  HV/1 -> Bus Creator/1  "HV_Vabc"
  LV/2 -> Bus Creator/4  "LV_Iabc"
  Bus Creator/1 -> m/1
  Open_Close_Breaker/1 -> Three-Phase Breaker/1
  Vabcref/1 -> Demux2/1
  Demux2/1 -> Controlled Voltage Source/1  "Va"
  Demux2/2 -> Controlled Voltage Source1/1  "Vb"
  Demux2/3 -> Controlled Voltage Source2/1  "Vc"
  connections:
  La_DVR1/LConn1 -- INV/RConn1
  LV/RConn1 -- Three-Phase Transformer (Two Windings)/RConn1 -- High Res Grounding/LConn1
  La_DVR1/RConn1 -- La_DVR4/RConn1 -- LV/LConn1
  Three-Phase Transformer (Two Windings)/LConn3 -- HV/LConn3
  Three-Phase Transformer (Two Windings)/RConn3 -- LV/RConn3 -- High Res Grounding/LConn3
  La_DVR2/RConn1 -- La_DVR5/RConn1 -- LV/LConn2
  Three-Phase Transformer (Two Windings)/LConn2 -- HV/LConn2
  Three-Phase Transformer (Two Windings)/RConn2 -- LV/RConn2 -- High Res Grounding/LConn2
  Three-Phase Transformer (Two Windings)/LConn1 -- HV/LConn1
  LV/LConn3 -- La_DVR3/RConn1 -- La_DVR6/RConn1
  La_DVR3/LConn1 -- INV/RConn3
  La_DVR5/LConn1 -- La_DVR6/LConn1 -- La_DVR4/LConn1
  La_DVR2/LConn1 -- INV/RConn2
  Three-Phase Breaker/LConn2 -- B/RConn1
  Three-Phase Breaker/RConn2 -- HV/RConn2
  HV/RConn3 -- Three-Phase Breaker/RConn3
  Three-Phase Breaker/LConn3 -- C/RConn1
  HV/RConn1 -- Three-Phase Breaker/RConn1
  Three-Phase Breaker/LConn1 -- A/RConn1
  Controlled Voltage Source2/LConn1 -- Controlled Voltage Source/LConn1 -- Controlled Voltage Source1/LConn1
  INV/LConn1 -- Controlled Voltage Source/RConn1
  Controlled Voltage Source1/RConn1 -- INV/LConn2
  Controlled Voltage Source2/RConn1 -- INV/LConn3

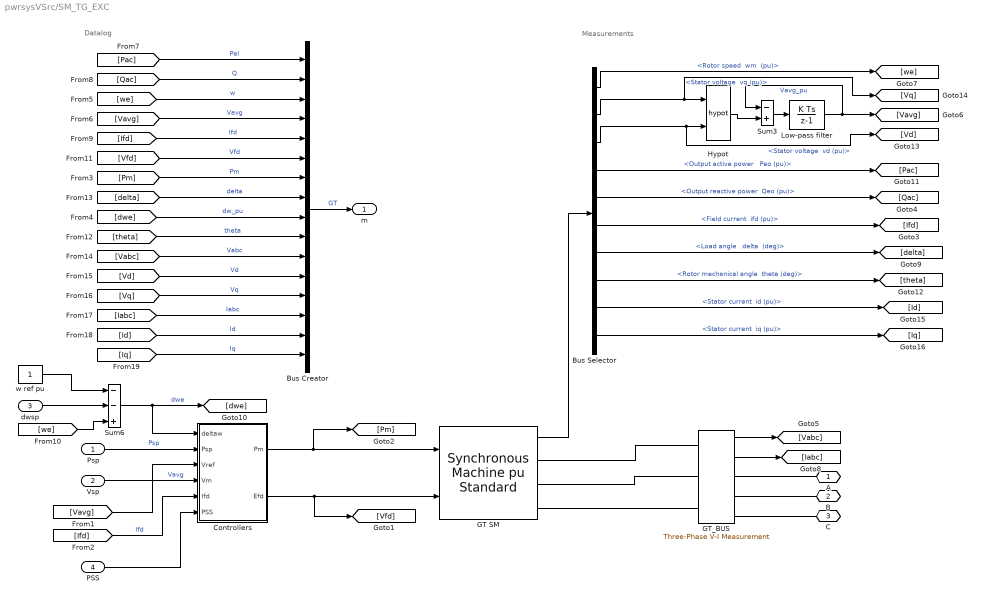
== system pwrsysVSrc/SM_TG_EXC ==
  note: Measurements
  note: Datalog
  Psp : Inport
  Vsp : Inport  Port=2
  dwsp : Inport  Port=3
  PSS : Inport  Port=4
  Bus Creator : BusCreator  Inputs=16
  Bus Selector : BusSelector  OutputSignals="Mechanical.Rotor speed  wm  (pu),dq0 components.Stator voltage  vq (pu),dq0 components.Stator voltage  vd (pu),Output active power   Peo (pu),Output reactive power  Qeo (pu),dq0 components.Field current  ifd (pu),Load angle   delta  (deg),Mechanical.Rotor mechanical angle  theta (deg),dq0 components.Stator current  id (pu),dq0 components.Stator current  iq (pu)"
  Controllers : Subsystem  SystemSampleTime=1/(20*grid.fn)
  GT SM : powerlib/Machines/Synchronous Machine pu Standard  PresetModel=No  MechanicalLoad=Mechanical power Pm  ShowDetailedParameters=on  RotorType=Salient-pole  Units=per unit standard parameters  MeasurementBus=off  NominalParameters=[SMPn SMVn SMfn]  Reactances1=[ 2.12, 0.299, 0.188, 1.76, 0.65, 0.25, 0.15 ]  Reactances2=[SMXd SMXdp SMXdpp SMXq SMXqpp SMXl]  dAxisTimeConstants=Short-circuit  qAxisTimeConstants=Short-circuit  TimeConstants1="[ 4.4849  0.0681  0.1  ]"  TimeConstants2=[ 8.0, 0.03, 1.0, 0.07 ]  TimeConstants3="[  4.49  0.0681  0.0513  ]"  TimeConstants4=[ 8.0, 0.03, 0.3371, 0.0295 ]  TimeConstants5=[ 1.01, 0.053, 0.1 ]  TimeConstants6=[ 1.3201, 0.023, 1.0, 0.07 ]  TimeConstants7=[SMTdpSC SMTdppSC SMTqppSC]  TimeConstants8=[ 1.3201, 0.0231, 0.3371, 0.0295 ]  StatorResistance=SMRs  Mechanical=[SMM 0 SMp]  PolePairs=20  InitialConditions=[SMdw0 SMth0 TurbP0/SMVt0 TurbP0/SMVt0 TurbP0/SMVt0 SMphi0 SMphi0-120 SMphi0+120 SMEfd0]  SetSaturation=on  Saturation=SMsat  LoadFlowParameters=[2 10000 0 0.1 0]  TsPowergui=0  TsBlock=-1  IterativeModel=Trapezoidal non iterative  IterativeDiscreteModel=Trapezoidal non iterative  BusType=swing  Pref=0  Qref=0  Qmin=-inf  Qmax=inf  PLF=0  QLF=0
  GT_BUS : powerlib/Measurements/Three-Phase V-I Measurement  VoltageMeasurement=phase-to-ground  SetLabelV=off  LabelV=vconv  Vpu=off  VpuLL=off  CurrentMeasurement=yes  SetLabelI=off  LabelI=iconv  Ipu=off  Pbase=sn  Vbase=uab  OutputType=Complex  PhasorSimulation=off  PSBequivalent=0
  Hypot : Math  Operator=hypot  SaturateOnIntegerOverflow=on
  Low-pass filter : DiscreteIntegrator  gainval=3/ExcTr  InitialCondition=SMVt0  InitialConditionSetting=State (most efficient)  SampleTime=Ts  UpperSaturationLimit=Refmax/Kp  LowerSaturationLimit=Refmin/Kp  ICPrevOutput=DiscIntNeverNeededParam  ICPrevScaledInput=DiscIntNeverNeededParam
  Sum3 : Sum  Inputs=-+
  Sum6 : Sum  Inputs=--+
  w ref pu : Constant  SampleTime=Ts
  A : PMIOPort  Port=1  Side=Right
  B : PMIOPort  Port=2  Side=Right
  C : PMIOPort  Port=3  Side=Right
  m : Outport
  wires:
  dwsp/1 -> Sum6/2
  [we] -> Sum6/3
  w ref pu/1 -> Sum6/1
  Bus Selector/6 -> [Ifd]  "<Field current  ifd (pu)>"
  GT SM/1 -> Bus Selector/1
  Bus Selector/5 -> [Qac]  "<Output reactive power  Qeo (pu)>"
  Bus Selector/3 -> [Vd], Hypot/2  "<Stator voltage  vd (pu)>"
  Bus Selector/2 -> [Vq], Hypot/1  "<Stator voltage  vq (pu)>"
  Bus Selector/1 -> [we]  "<Rotor speed  wm  (pu)>"
  Bus Selector/4 -> [Pac]  "<Output active power   Peo (pu)>"
  [Vavg] -> Bus Creator/4  "Vavg"
  [Pac] -> Bus Creator/1  "Pel"
  [Qac] -> Bus Creator/2  "Q"
  [we] -> Bus Creator/3  "w"
  [Ifd] -> Bus Creator/5  "Ifd"
  [Vfd] -> Bus Creator/6  "Vfd"
  Bus Creator/1 -> m/1  "GT"
  Sum6/1 -> Controllers/1(deltaw), [dwe]  "dwe"
  Psp/1 -> Controllers/2(Psp)  "Psp"
  Vsp/1 -> Controllers/3(Vref)
  [Vavg] -> Controllers/4(Vm)  "Vavg"
  [Ifd] -> Controllers/5(Ifd)  "Ifd"
  [Pm] -> Bus Creator/7  "Pm"
  Controllers/2(Efd) -> [Vfd], GT SM/2
  Controllers/1(Pm) -> [Pm], GT SM/1
  Low-pass filter/1 -> [Vavg], Sum3/1  "Vavg_pu"
  Sum3/1 -> Low-pass filter/1
  Hypot/1 -> Sum3/2
  GT_BUS/1 -> [Vabc]
  GT_BUS/2 -> [Iabc]
  Bus Selector/7 -> [delta]  "<Load angle   delta  (deg)>"
  Bus Selector/8 -> [theta]  "<Rotor mechanical angle  theta (deg)>"
  [theta] -> Bus Creator/10  "theta"
  [dwe] -> Bus Creator/9  "dw_pu"
  [delta] -> Bus Creator/8  "delta"
  PSS/1 -> Controllers/6(PSS)
  [Vabc] -> Bus Creator/11  "Vabc"
  [Vd] -> Bus Creator/12  "Vd"
  [Vq] -> Bus Creator/13  "Vq"
  [Iabc] -> Bus Creator/14  "Iabc"
  [Id] -> Bus Creator/15  "Id"
  [Iq] -> Bus Creator/16  "Iq"
  Bus Selector/9 -> [Id]  "<Stator current  id (pu)>"
  Bus Selector/10 -> [Iq]  "<Stator current  iq (pu)>"
  connections:
  B/RConn1 -- GT_BUS/RConn2
  A/RConn1 -- GT_BUS/RConn1
  C/RConn1 -- GT_BUS/RConn3
  GT_BUS/LConn1 -- GT SM/RConn1
  GT_BUS/LConn2 -- GT SM/RConn2
  GT_BUS/LConn3 -- GT SM/RConn3

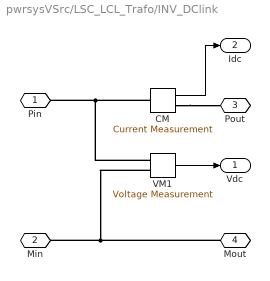
== system pwrsysVSrc/LSC_LCL_Trafo/INV_DClink ==
  CM : powerlib/Measurements/Current Measurement  PhasorSimulation=off  OutputType=Complex  PSBequivalent=0
  VM1 : powerlib/Measurements/Voltage Measurement  PhasorSimulation=off  OutputType=Complex  PSBequivalent=0
  Pin : PMIOPort  Port=1  Side=Left
  Min : PMIOPort  Port=2  Side=Left
  Pout : PMIOPort  Port=3  Side=Right
  Mout : PMIOPort  Port=4  Side=Right
  Vdc : Outport
  Idc : Outport  Port=2
  wires:
  CM/1 -> Idc/1
  VM1/1 -> Vdc/1
  connections:
  VM1/LConn2 -- Mout/RConn1 -- Min/RConn1
  VM1/LConn1 -- CM/LConn1 -- Pin/RConn1
  CM/RConn1 -- Pout/RConn1

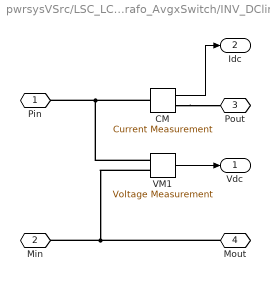
== system pwrsysVSrc/LSC_LCL_Trafo_AvgxSwitch/INV_DClink ==
  CM : powerlib/Measurements/Current Measurement  PhasorSimulation=off  OutputType=Complex  PSBequivalent=0
  VM1 : powerlib/Measurements/Voltage Measurement  PhasorSimulation=off  OutputType=Complex  PSBequivalent=0
  Pin : PMIOPort  Port=1  Side=Left
  Min : PMIOPort  Port=2  Side=Left
  Pout : PMIOPort  Port=3  Side=Right
  Mout : PMIOPort  Port=4  Side=Right
  Vdc : Outport
  Idc : Outport  Port=2
  wires:
  CM/1 -> Idc/1
  VM1/1 -> Vdc/1
  connections:
  VM1/LConn2 -- Mout/RConn1 -- Min/RConn1
  VM1/LConn1 -- CM/LConn1 -- Pin/RConn1
  CM/RConn1 -- Pout/RConn1

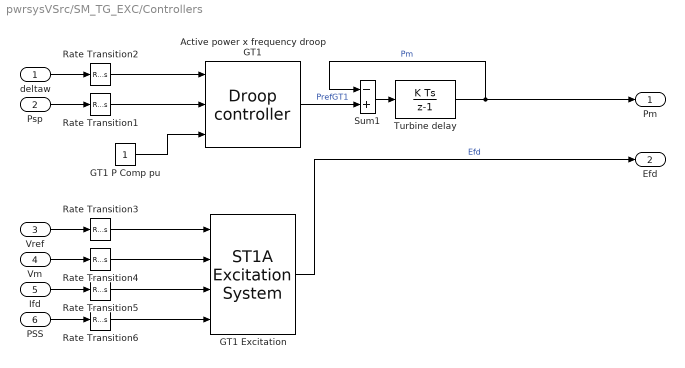
== system pwrsysVSrc/SM_TG_EXC/Controllers ==
  deltaw : Inport
  Psp : Inport  Port=2
  Vref : Inport  Port=3
  Vm : Inport  Port=4
  Ifd : Inport  Port=5
  PSS : Inport  Port=6
  Active power x frequency droop GT1 : pwrsysBasic/Droop controller  Refmax=SMcosphi  Refmin=0  Ts=Ts  Kp=GovKp  Kd=GovKd  Tr=GovTr  flp=GovFlp  DB=GovDB
  GT1 Excitation : sps_avr/ST1A Excitation System  Tr=ExcTr  KaTa=[ExcKa 1/(6*SMfn)]  VIminmax=[-0.2 0.2]  VAminmax=[ExcVRMin ExcVRMax]  VRminmax=[ExcVRMin ExcVRMax]  KfTf=[ExcKf ExcTf]  TbTc=[ExcTb ExcTc ExcTb1 ExcTc1]  KLR=0  ILR=999  Kc=0  v0=[SMVt0,sqrt(2/3)*SMEfd0]  TsBlock=Ts
  GT1 P Comp pu : Constant  SampleTime=-1
  Rate Transition{1..6} (6 alike) : RateTransition  OutPortSampleTime=Ts
  Sum1 : Sum  Inputs=-+
  Turbine delay : DiscreteIntegrator  gainval=1/TurbT  InitialCondition=TurbP0  InitialConditionSetting=State (most efficient)  SampleTime=Ts  LimitOutput=on  UpperSaturationLimit=SMcosphi  LowerSaturationLimit=0  ICPrevOutput=DiscIntNeverNeededParam  ICPrevScaledInput=DiscIntNeverNeededParam
  Pm : Outport
  Efd : Outport  Port=2
  wires:
  Vref/1 -> Rate Transition3/1
  Vm/1 -> Rate Transition4/1
  Active power x frequency droop GT1/1 -> Sum1/2  "PrefGT1"
  Rate Transition6/1 -> GT1 Excitation/4
  Turbine delay/1 -> Pm/1, Sum1/1  "Pm"
  GT1 Excitation/1 -> Efd/1  "Efd"
  GT1 P Comp pu/1 -> Active power x frequency droop GT1/3
  Ifd/1 -> Rate Transition5/1
  Sum1/1 -> Turbine delay/1
  Psp/1 -> Rate Transition1/1
  deltaw/1 -> Rate Transition2/1
  Rate Transition2/1 -> Active power x frequency droop GT1/1
  Rate Transition1/1 -> Active power x frequency droop GT1/2
  Rate Transition3/1 -> GT1 Excitation/1
  Rate Transition4/1 -> GT1 Excitation/2
  Rate Transition5/1 -> GT1 Excitation/3
  PSS/1 -> Rate Transition6/1
